simulink model "UAV_MPC_Tracking2D"  (R2025b)
settings: Solver=ode4  StartTime=0.0  StopTime=120  FixedStep=Ts  RelTol=1e-3
InitFcn:
  | initMPC
undefined symbols (not defined in the file): start, trajXY
libraries: mpclib x1
settings Model: Creator=EBIRON  LastModifiedBy=EBIRON

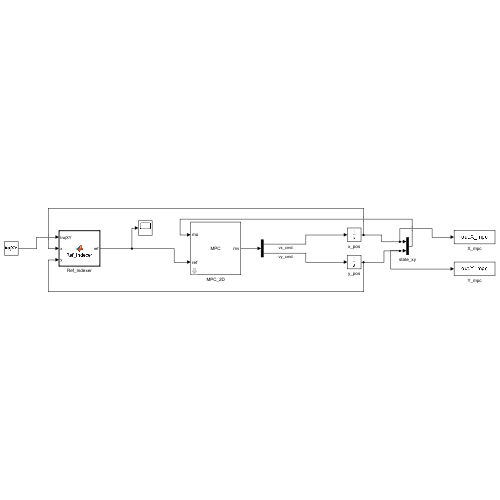
[thumbnail: Simulink's stored preview of the top-level diagram]
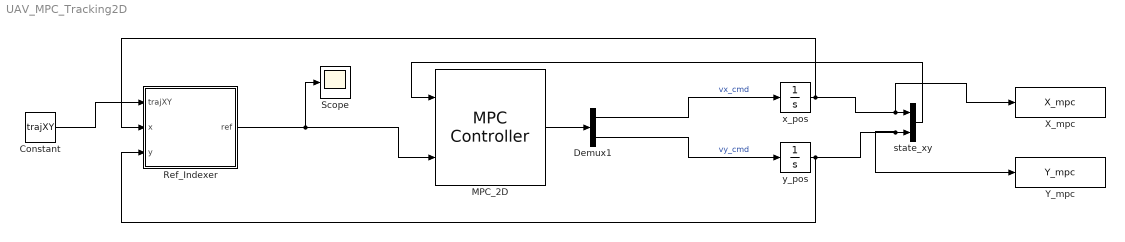
== system UAV_MPC_Tracking2D ==
  Constant : Constant  Value=trajXY  OutDataTypeStr=double
  Demux1 : Demux  Outputs=2
  MPC_2D : mpclib/MPC Controller  SCDEnableBlockLinearizationSpecification=on  mpcobj=mpcobj  is_multiple=0  enable_value=0  return_u0=off  updateMPCinCallerWorkspace=on  md_inport=off  mv_inport=off  uref_inport=off  return_cost=off  return_mvseq=off  return_qpstatus=off  return_xseq=off  return_state=off  return_ovseq=off  state_inport=off  umin_inport=off  umax_inport=off  ymin_inport=off  ymax_inport=off  cc_inport=off  ywt_inport=off  uwt_inport=off  duwt_inport=off  rhoeps_inport=off  pm_inport=off  MaximumP=10  HorizonChoice=FixedHorizon  n_ts=0.1  n_p=40  n_mv=2  n_md=0  n_ud=0  n_mo=2  n_uo=0  BlockDataType=double  SampleTimeInherited=off  switch_inport=off
  "Ref_Indexer " : MATLAB Function  TreatAsAtomicUnit=on
  Scope : Scope
      settings: ActiveDisplayYMinimum=-1  ActiveDisplayYMaximum=1
  X_mpc : ToWorkspace  VariableName=X_mpc  SampleTime=-1
  Y_mpc : ToWorkspace  VariableName=Y_mpc  SampleTime=-1
  state_xy : Mux  Inputs=2
  x_pos : Integrator  InitialCondition=start(1)
  y_pos : Integrator  InitialCondition=start(2)
  wires:
  Demux1/1 -> x_pos/1  "vx_cmd"
  Demux1/2 -> y_pos/1  "vy_cmd"
  x_pos/1 -> "Ref_Indexer "/2(x), X_mpc/1, state_xy/1
  y_pos/1 -> "Ref_Indexer "/3(y), state_xy/2, Y_mpc/1
  state_xy/1 -> MPC_2D/1
  MPC_2D/1 -> Demux1/1
  Constant/1 -> "Ref_Indexer "/1(trajXY)
  "Ref_Indexer "/1(ref) -> Scope/1, MPC_2D/2

== matlab function UAV_MPC_Tracking2D/Ref_Indexer  ==
  settings: updateMethod=DISCRETE  sampleTime=0.1
  data: trajXY input; ref output double size=[1 2]; x input; y input
function ref = Ref_Indexer(trajXY, x, y)
% trajXY : [N x 2] constant path
% x, y   : current UAV position

%#codegen

% Persistent index memory
persistent idx_prev
if isempty(idx_prev)
    idx_prev = 1;
end

% Path length (compile-time constant)
N = coder.const(size(trajXY,1));

% Find nearest point
minDist = 1e12;
idx_near = idx_prev;

for i = idx_prev:N   % IMPORTANT: start from previous index
    dx = trajXY(i,1) - x;
    dy = trajXY(i,2) - y;
    d2 = dx*dx + dy*dy;

    if d2 < minDist
        minDist = d2;
        idx_near = i;
    end
end

% Enforce forward progress
if idx_near < idx_prev
    idx_near = idx_prev;
end

% Lookahead
lookahead = 5;
idx_ref = idx_near + lookahead;

if idx_ref > N
    idx_ref = N;
end

% Update memory
idx_prev = idx_near;

% Output reference
ref = trajXY(idx_ref,:);
end
